simulink library "CompatHash"  (R2022b)
settings: Solver=VariableStepAuto  StartTime=0.0  StopTime=10.0  RelTol=1e-3
libraries: HandyTextFile x1, ITC x1, StateVar x1
settings Model: Creator=kl13806  LastModifiedBy=kl13806
settings SolverCC: AlgebraicLoopSolver=TrustRegion
settings DebuggingCC: UnconnectedInputMsg=warning  UnconnectedOutputMsg=warning  UnconnectedLineMsg=warning  SFMachineParentedDataDiag=warning
settings ModelReferenceCC: EnableRefExpFcnMdlSchedulingChecks=on
settings RTWCC: DLArmComputeVersion=19.05

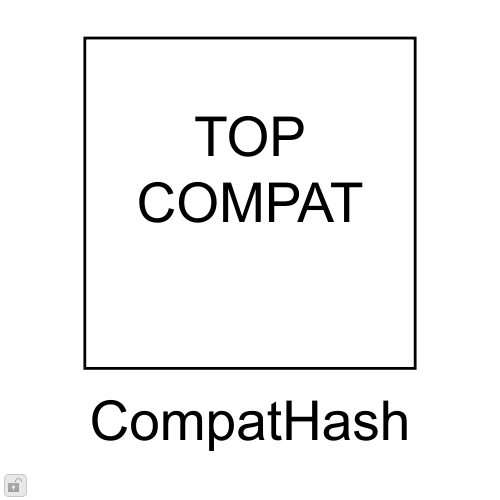
[thumbnail: Simulink's stored preview of the top-level diagram]
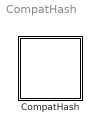
== system CompatHash ==
  CompatHash : Subsystem  mask(Talaria Compat Block){CompatType=TOP: COMPAT code for Target Overlay Parameter tokens}
      mask help: This block surfaces a TargetStateVar (i.e. StateVar and TSP) that returns the COMPAT hash code for a set of tokens. Since this hash code is computed by looking at all partitioned cores, a valid value is not achieved unless the official partitioning tool scripts are used. Choose the token set below
      mask init:
      | blkh = gcbh;
      | groupPath = CompatHashMask.DoInit(blkh, CompatType);
      mask TypeOptions CompatType: TOP: COMPAT code for Target Overlay Parameter tokens | TSP: COMPAT code for Target State Probe tokens
      mask DialogControl TextLabel Prompt: Overlay Group:
      mask DialogControl TextOverlayPath Prompt: (Add text here)
      mask Display:
      | disp( [...
      |     CompatHashMask.cfg(CompatType).blockType newline ...
      |     'COMPAT' newline ...
      |     groupPath]);

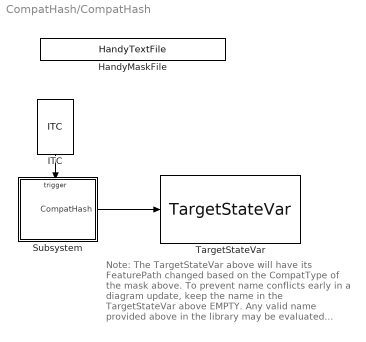
== system CompatHash/CompatHash ==
  note: Note: The TargetStateVar above will have its FeaturePath changed based on the CompatType of the mask above. To prevent name conflicts early in a diagram update, keep the name in the TargetStateVar above EMPTY. Any valid name provided above in the library may be evaluated before the mask magic completes, leading to name conflicts.
  HandyMaskFile : HandyTextFile/HandyTextFile  TemplateSource=Mask  FileSuffix=Init  OpenDialogOnLoad=off  UseThisBlockName=off  TheDefaultText=|  ShowInLibBrowser=on
      | % $(FILENAME) Setup model parameters for each "Init" callback (e.g. update diagram)
      | sample_rate_in_hertz = 44100;
      | frame_size = 32;
      | sysin_channel_count = 2;
      settings: SourceProductName=Bose Talaria
  ITC : ITC/ITC
      settings: SourceProductName=Bose Talaria
  Subsystem : Subsystem
      settings: RTWSystemCode=Inline
  TargetStateVar : StateVar/TargetStateVar  TriggerInit=[185 6 325 74]  UseSameName=on  IfdefMacro='CAPTURE_CONSTANT_TSPS'
      settings: SourceProductName=Bose Talaria
  wires:
  Subsystem/1(CompatHash) -> TargetStateVar/1
  ITC/1 -> Subsystem/Trigger

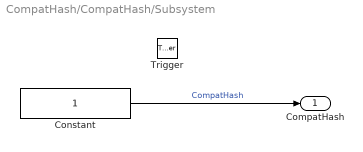
== system CompatHash/CompatHash/Subsystem ==
  Trigger : TriggerPort  TriggerType=function-call  VariantControl=Variant  PortDimensions=1
  Constant : Constant  SampleTime=-1
  CompatHash : Outport
  wires:
  Constant/1 -> CompatHash/1  "CompatHash"
